simulink model "Cv_2_fsi"  (R2022a)
settings: Solver=VariableStepAuto  StartTime=0  StopTime=2  RelTol=1e-6
settings Model: Creator=221208  LastModifiedBy=221208

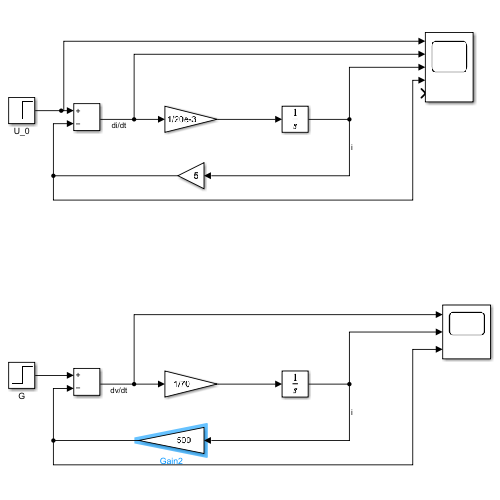
[thumbnail: Simulink's stored preview of the top-level diagram]
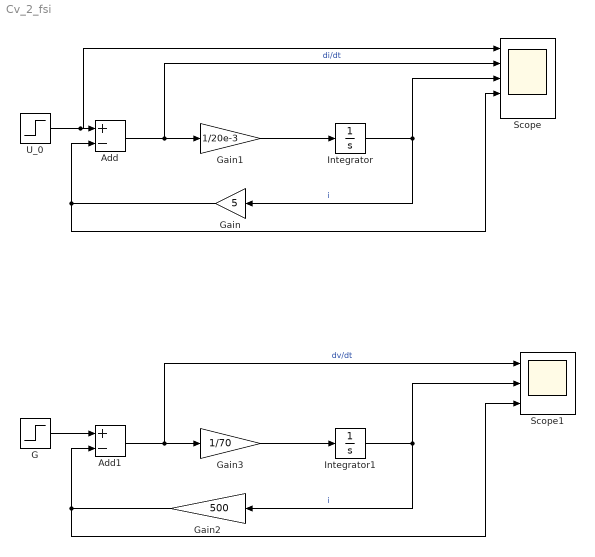
== system Cv_2_fsi ==
  Add : Sum  Inputs=+-
  Add1 : Sum  Inputs=+-
  G : Step  After=70  SampleTime=0
  Gain : Gain  Gain=5
  Gain1 : Gain  Gain=1/20e-3
  Gain2 : Gain  Gain=500
  Gain3 : Gain  Gain=1/70
  Integrator : Integrator
  Integrator1 : Integrator
  Scope : Scope  NumInputPorts=5
  Scope1 : Scope  NumInputPorts=3
  U_0 : Step  After=12  SampleTime=0
  wires:
  Add/1 -> Scope/2, Gain1/1  "di/dt"
  U_0/1 -> Scope/1, Add/1
  Integrator/1 -> Scope/3, Gain/1  "i"
  Gain/1 -> Scope/4, Add/2
  Gain1/1 -> Integrator/1
  Gain3/1 -> Integrator1/1
  Add1/1 -> Scope1/1, Gain3/1  "dv/dt"
  Gain2/1 -> Scope1/3, Add1/2
  Integrator1/1 -> Scope1/2, Gain2/1  "i"
  G/1 -> Add1/1
